simulink model "MIMOcontroller2020a"  (R2020a)
settings: Solver=ode4  StartTime=0.0  StopTime=5  FixedStep=0.01  RelTol=1e-3  EnableMultiTasking=on
undefined symbols (not defined in the file or in its folder): den11, den12, den21, den22, den_d11, den_d12, den_d21, den_d22, den_gc1, den_gc2, den_h11, den_h22, num11, num12, num21, num22, num_d11, num_d12, num_d21, num_d22, num_gc1, num_gc2, num_h11, num_h22
settings Model: Creator=alexandra  LastModifiedBy=alexandra
settings DataIOCC: LimitDataPoints=on  SaveFormat=Array  ReturnWorkspaceOutputs=off
settings OptimizationCC: LifeSpan=inf
settings DebuggingCC: SFUnexpectedBacktrackingDiag=warning  SFNoUnconditionalDefaultTransitionDiag=warning  SFExecutionAtInitializationDiag=none  ArithmeticOperatorsInVariantConditions=warning
settings HardwareCC: ProdBitPerPointer=32  ProdBitPerSizeT=32  ProdBitPerPtrDiffT=32  ProdLargestAtomicFloat=None  ProdIntDivRoundTo=Undefined  ProdEndianess=Unspecified  ProdWordSize=32  ProdHWDeviceType=32-bit Generic
settings ModelReferenceCC: PropagateSignalLabelsOutOfModel=off
settings SFSimCC: SimUseLocalCustomCode=off  CustomCodeUndefinedFunction=UseInterfaceOnly
settings RTWCC: RTWUseLocalCustomCode=off
settings CodeAppCC: StateflowObjectComments=on
settings GRTTargetCC: TargetLangStandard=C89/C90 (ANSI)
settings ConfigComp: CovMetricSettings=dw  CovSaveCumulativeToWorkspaceVar=on  CovSaveSingleToWorkspaceVar=on  CovExternalEMLEnable=off

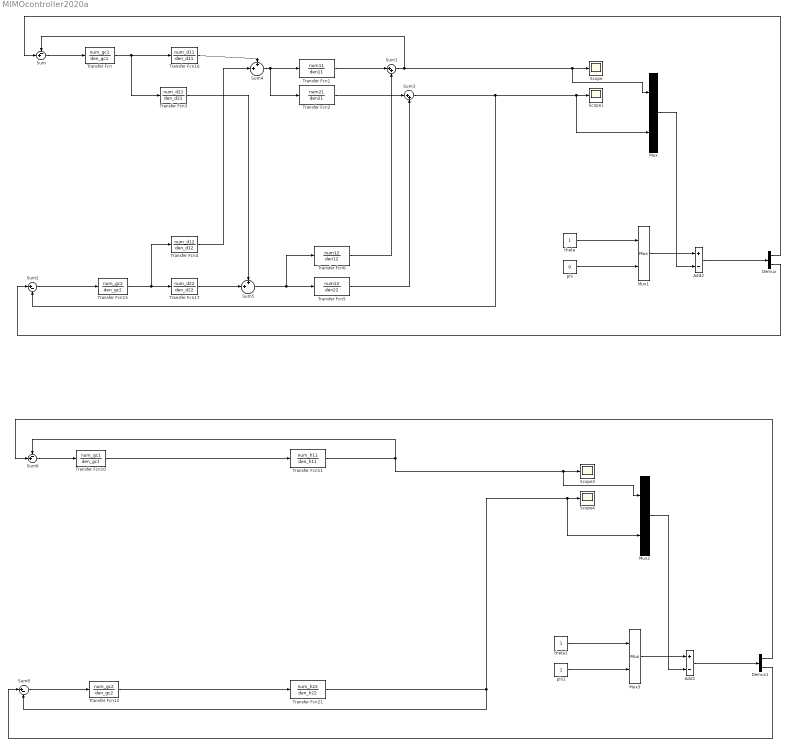
== system MIMOcontroller2020a ==
  Add1 : Sum  Inputs=+-
  Add2 : Sum  Inputs=+-
  Demux : Demux  Outputs=2
  Demux1 : Demux  Outputs=2
  Mux{,1..3} (4 alike) : Mux  Inputs=2
  Scope{,1,3..4} (4 alike) : Scope
  Sum : Sum  Inputs=-+|
  Sum1 : Sum  Inputs=|++
  Sum2 : Sum  Inputs=|+-
  Sum3 : Sum  Inputs=|++
  Sum4 : Sum  Inputs=++|
  Sum5 : Sum  Inputs=++|
  Sum6 : Sum  Inputs=-+|
  Sum8 : Sum  Inputs=|+-
  Transfer Fcn : TransferFcn  Numerator=num_gc1  Denominator=den_gc1
  Transfer Fcn1 : TransferFcn  Numerator=num11  Denominator=den11
  Transfer Fcn10 : TransferFcn  Numerator=num_gc1  Denominator=den_gc1
  Transfer Fcn11 : TransferFcn  Numerator=num_h11  Denominator=den_h11
  Transfer Fcn12 : TransferFcn  Numerator=num_gc2  Denominator=den_gc2
  Transfer Fcn15 : TransferFcn  Numerator=num_gc2  Denominator=den_gc2
  Transfer Fcn16 : TransferFcn  Numerator=num_d11  Denominator=den_d11
  Transfer Fcn17 : TransferFcn  Numerator=num_d22  Denominator=den_d22
  Transfer Fcn2 : TransferFcn  Numerator=num21  Denominator=den21
  Transfer Fcn21 : TransferFcn  Numerator=num_h22  Denominator=den_h22
  Transfer Fcn3 : TransferFcn  Numerator=num_d21  Denominator=den_d21
  Transfer Fcn4 : TransferFcn  Numerator=num_d12  Denominator=den_d12
  Transfer Fcn5 : TransferFcn  Numerator=num22  Denominator=den22
  Transfer Fcn6 : TransferFcn  Numerator=num12  Denominator=den12
  phi : Constant  Value=0
  phi1 : Constant
  theta : Constant
  theta1 : Constant
  wires:
  Sum4/1 -> Transfer Fcn1/1, Transfer Fcn2/1
  Transfer Fcn15/1 -> Transfer Fcn4/1, Transfer Fcn17/1
  Sum5/1 -> Transfer Fcn6/1, Transfer Fcn5/1
  Transfer Fcn1/1 -> Sum1/1
  Sum1/1 -> Sum/1, Mux/1, Scope/1
  Sum/1 -> Transfer Fcn/1
  Sum2/1 -> Transfer Fcn15/1
  theta/1 -> Mux1/1
  Mux1/1 -> Add2/1
  Mux/1 -> Add2/2
  Transfer Fcn5/1 -> Sum3/2
  Add2/1 -> Demux/1
  Transfer Fcn/1 -> Transfer Fcn3/1, Transfer Fcn16/1
  Transfer Fcn16/1 -> Sum4/1
  Transfer Fcn17/1 -> Sum5/2
  Demux/1 -> Sum/2
  Demux/2 -> Sum2/1
  Sum3/1 -> Sum2/2, Scope1/1, Mux/2
  phi/1 -> Mux1/2
  Transfer Fcn3/1 -> Sum5/1
  Transfer Fcn4/1 -> Sum4/2
  Transfer Fcn6/1 -> Sum1/2
  Transfer Fcn2/1 -> Sum3/1
  Demux1/2 -> Sum8/1
  phi1/1 -> Mux3/2
  theta1/1 -> Mux3/1
  Mux2/1 -> Add1/2
  Mux3/1 -> Add1/1
  Transfer Fcn21/1 -> Scope4/1, Mux2/2, Sum8/2
  Demux1/1 -> Sum6/2
  Add1/1 -> Demux1/1
  Sum6/1 -> Transfer Fcn10/1
  Sum8/1 -> Transfer Fcn12/1
  Transfer Fcn12/1 -> Transfer Fcn21/1
  Transfer Fcn10/1 -> Transfer Fcn11/1
  Transfer Fcn11/1 -> Mux2/1, Scope3/1, Sum6/1
